simulink model "Multi_agent_system"  (R2016b)
settings: Solver=VariableStepAuto  StartTime=0.0  StopTime=10  RelTol=1e-3
undefined symbols (not defined in the file or in its folder): A, B, Kr, Kv, n, v_initial, x_initial
settings Model: Creator=kvlton  LastModifiedBy=kvlton

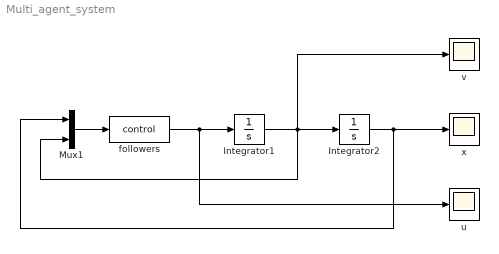
== system Multi_agent_system ==
  Integrator1 : Integrator  InitialCondition=v_initial
  Integrator2 : Integrator  InitialCondition=x_initial
  Mux1 : Mux  Inputs=2
  followers : S-Function  FunctionName=control  Parameters=A,B,n,Kr,Kv  SFunctionDeploymentMode=off  EnableBusSupport=off
  u : Scope
  v : Scope
  x : Scope
  wires:
  Mux1/1 -> followers/1
  followers/1 -> u/1, Integrator1/1
  Integrator1/1 -> Mux1/2, v/1, Integrator2/1
  Integrator2/1 -> Mux1/1, x/1
